simulink model "Practice_and_Demo"  (R2024b)
settings: Solver=FixedStepAuto  StartTime=0.0  StopTime=inf  RelTol=1e-3  EnableMultiTasking=on
libraries: spsabctodq0Lib x1
settings Model: Creator=mafur  LastModifiedBy=mafur
settings SolverCC: PositivePriorityOrder=on
settings OptimizationCC: DefaultParameterBehavior=Inlined  DefaultUnderspecifiedDataType=single  EnhancedBackFolding=on  PassReuseOutputArgsAs=Individual arguments  ZeroExternalMemoryAtStartup=off  MaxStackSize=200000  OptimizeBlockOrder=speed  DifferentSizesBufferReuse=on  OptimizationCustomize=off  EfficientTunableParamExpr=on
settings DebuggingCC: ParameterTunabilityLossMsg=error
settings HardwareCC: ProdBitPerPointer=32  ProdBitPerSizeT=32  ProdBitPerPtrDiffT=32  ProdLargestAtomicInteger=Long  ProdLargestAtomicFloat=Double  ProdWordSize=32  ProdLongLongMode=on  ProdHWDeviceType=ARM Compatible->ARM Cortex-A (32-bit)
settings RTWCC: Description=Embedded Coder  SystemTargetFile=ert.tlc  HardwareBoard=Raspberry Pi  TLCOptions="-aInlineSetEventsForThisBaseRateFcn=TLC_FALSE -aSuppressMultiTaskScheduler=TLC_FALSE  -aRateBasedStepFcn=0"  TemplateMakefile=ert_default_tmf  Toolchain=GNU GCC Embedded Linux  BuildConfiguration=Faster Runs
settings CodeAppCC: ForceParamTrailComments=on  IgnoreCustomStorageClasses=off  OperatorAnnotations=on  SimulinkDataObjDesc=on  SFDataObjDesc=on  InsertBlockDesc=on
settings ERTTargetCC: CodeReplacementLibrary=ARM Cortex-A CMSIS  SupportVariableSizeSignals=on  ExtModeTransport=2  ExtModeStaticAlloc=on  ExtModeMexFile=ext_xcp  ExtModeIntrfLevel=Level2 - Open

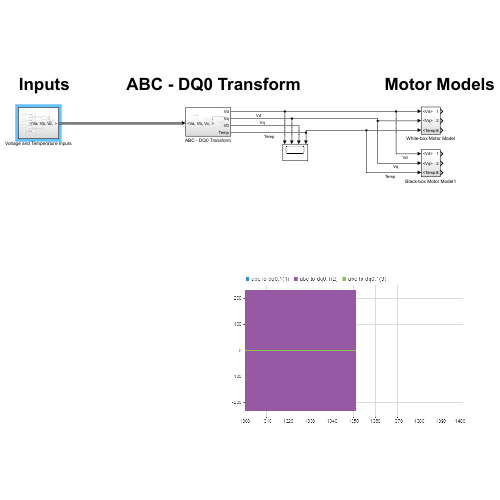
[thumbnail: Simulink's stored preview of the top-level diagram]
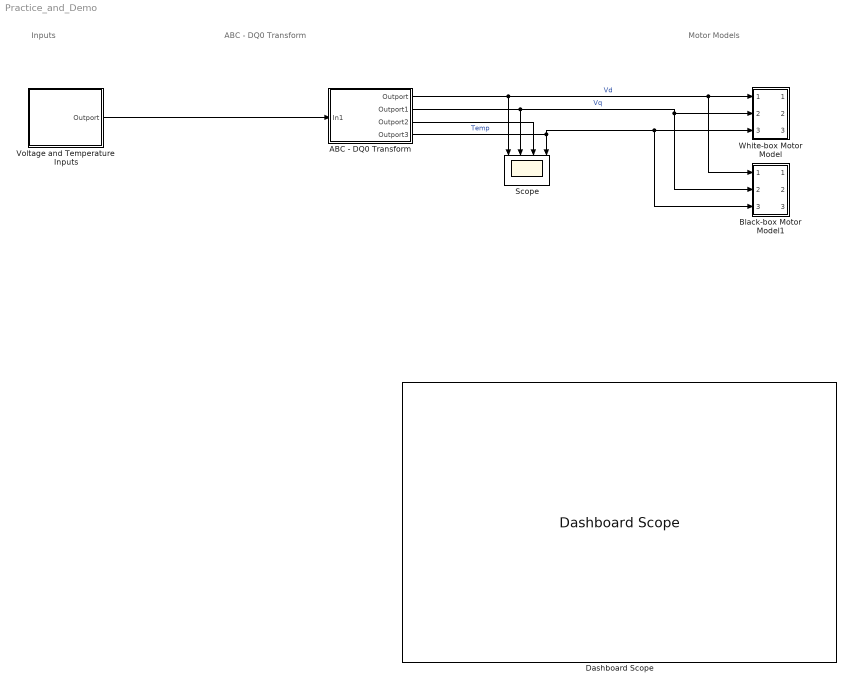
== system Practice_and_Demo ==
  note: Inputs
  note: ABC - DQ0 Transform
  note: Motor Models
  ABC - DQ0 Transform : Subsystem
  Black-box Motor Model1 : Subsystem
  Dashboard Scope : DashboardScope
  Scope : Scope  NumInputPorts=4
  Voltage and Temperature Inputs : Subsystem
  White-box Motor Model : Subsystem
  wires:
  Voltage and Temperature Inputs/1(Outport) -> ABC - DQ0 Transform/1(In1)
  ABC - DQ0 Transform/1(Outport) -> Scope/1, Black-box Motor Model1/1(Inport), White-box Motor Model/1(Inport)  "Vd"
  ABC - DQ0 Transform/2(Outport1) -> Scope/2, Black-box Motor Model1/2(Inport1), White-box Motor Model/2(Inport1)  "Vq"
  ABC - DQ0 Transform/3(Outport2) -> Scope/3
  ABC - DQ0 Transform/4(Outport3) -> Black-box Motor Model1/3(Inport2), White-box Motor Model/3(Inport2), Scope/4  "Temp"

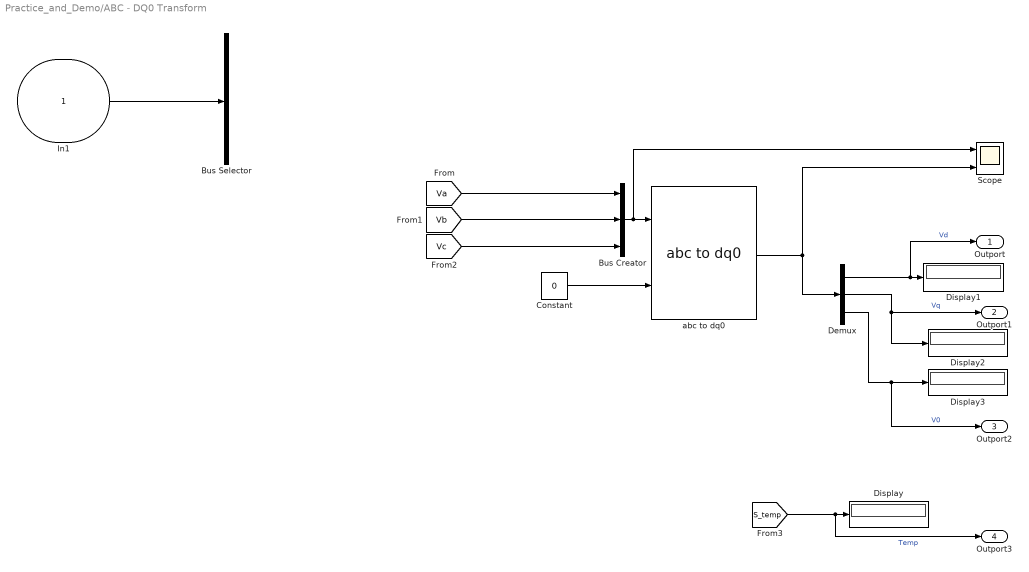
== system Practice_and_Demo/ABC - DQ0 Transform ==
  In1 : Inport
  Bus Creator : BusCreator  Inputs=3
  Bus Selector : BusSelector  OutputSignals=Va,Vb,Vc,signal4
  Constant : Constant  Value=0
  Demux : Demux  Outputs=3
  Display{,1..3} (4 alike) : Display
  Scope : Scope  NumInputPorts=2
  abc to dq0 : spsabctodq0Lib/abc to dq0  Alignment=Aligned with phase A axis
  Outport : Outport
  Outport1 : Outport  Port=2
  Outport2 : Outport  Port=3
  Outport3 : Outport  Port=4
  wires:
  Constant/1 -> abc to dq0/2
  [S_temp] -> Outport3/1, Display/1  "Temp"
  abc to dq0/1 -> Demux/1, Scope/2
  Bus Creator/1 -> Scope/1, abc to dq0/1
  Demux/2 -> Outport1/1, Display2/1  "Vq"
  Demux/3 -> Outport2/1, Display3/1  "V0"
  [Vb] -> Bus Creator/2
  [Vc] -> Bus Creator/3
  [Va] -> Bus Creator/1
  Demux/1 -> Outport/1, Display1/1  "Vd"
  In1/1 -> Bus Selector/1

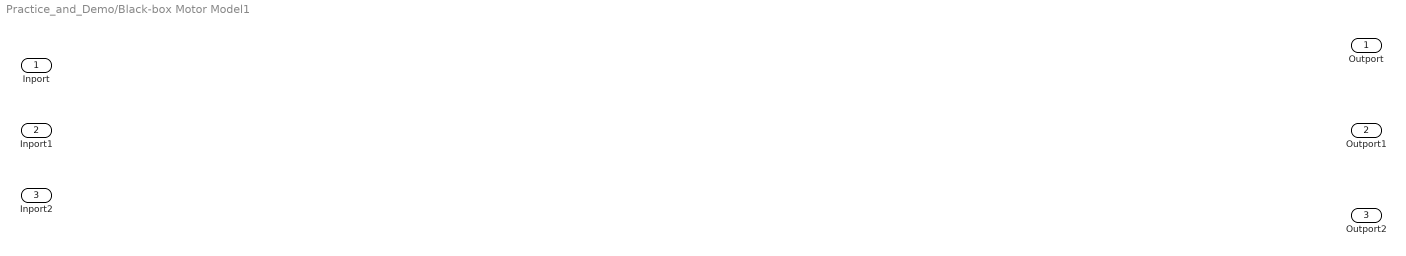
== system Practice_and_Demo/Black-box Motor Model1 ==
  Inport : Inport
  Inport1 : Inport  Port=2
  Inport2 : Inport  Port=3
  Outport : Outport
  Outport1 : Outport  Port=2
  Outport2 : Outport  Port=3

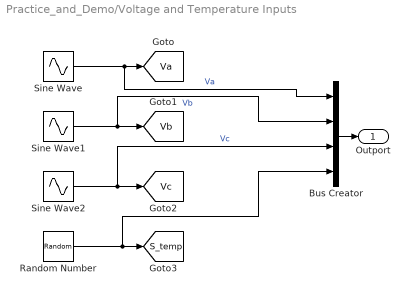
== system Practice_and_Demo/Voltage and Temperature Inputs ==
  Bus Creator : BusCreator  Inputs=4
  Random Number : RandomNumber  Mean=30  SampleTime=0.001
  Sine Wave : Sin  Amplitude=230  Frequency=314.16  SampleTime=0.001
  Sine Wave1 : Sin  Amplitude=230  Frequency=314.16  Phase=(2*pi)/3  SampleTime=0.001
  Sine Wave2 : Sin  Amplitude=230  Frequency=314.16  Phase=-(2*pi)/3  SampleTime=0.001
  Outport : Outport
  tag scope: S_temp=global, Va=global, Vb=global, Vc=global
  wires:
  Random Number/1 -> Bus Creator/4, [S_temp]
  Sine Wave1/1 -> Bus Creator/2, [Vb]  "Vb"
  Sine Wave2/1 -> Bus Creator/3, [Vc]  "Vc"
  Sine Wave/1 -> Bus Creator/1, [Va]  "Va"
  Bus Creator/1 -> Outport/1

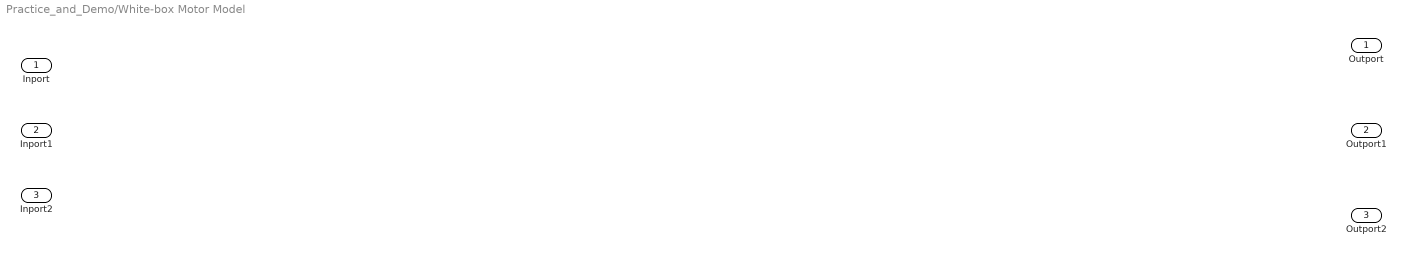
== system Practice_and_Demo/White-box Motor Model ==
  Inport : Inport
  Inport1 : Inport  Port=2
  Inport2 : Inport  Port=3
  Outport : Outport
  Outport1 : Outport  Port=2
  Outport2 : Outport  Port=3
